simulink model "simu_21uec072"  (R2022b)
settings: Solver=VariableStepAuto  StartTime=0.0  StopTime=0  RelTol=1e-3
settings Model: Creator=DSP-35  LastModifiedBy=DSP-35

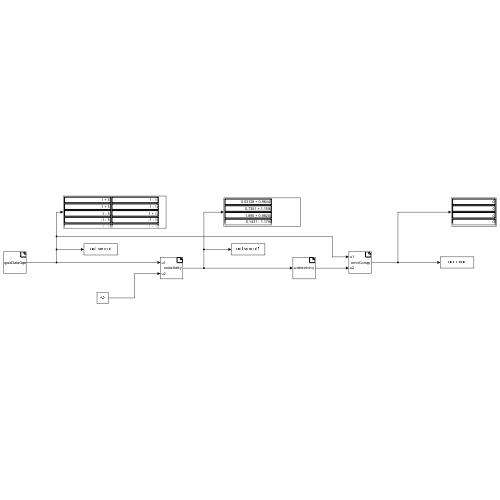
[thumbnail: Simulink's stored preview of the top-level diagram]
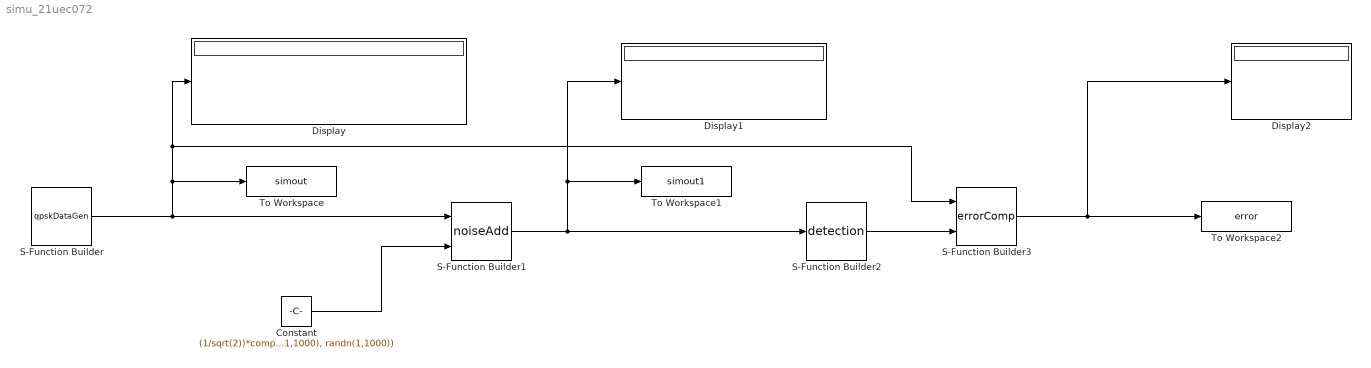
== system simu_21uec072 ==
  Constant : Constant  Value=(1/sqrt(2))*complex(randn(1,1000), randn(1,1000))
  Display : Display
  Display1 : Display
  Display2 : Display
  S-Function Builder : S-Function  FunctionName=qpskDataGen  SFunctionModules=qpskDataGen_wrapper.c  SFunctionDeploymentMode=off  EnableBusSupport=off  mask(S-Function Builder){}
      mask help: Simulink:masks:SFunctionBuilder_MD
      mask init:
      | val = [[.9  0.75 0.75 1 1 .9 .9 1]',[1 1 0.75 0.75 .9 .9 1 .9]'];try , sys = get_param(gcb,'SfunBuilderFcnName');if isempty(sys), sys = get_param(gcb,'FunctionName'); end,catch, sys = get_param(gcb,'FunctionName'); end
      settings: CopyFcn=set_param(gcbh,'LinkStatus','none')  OpenFcn=sfunctionwizard(gcbh)
      mask Display:
      | plot(val(:,1),val(:,2))
      | disp(sys)
      | port_label('output',1,'y')
  S-Function Builder1 : S-Function  FunctionName=noiseAdd  SFunctionModules=noiseAdd_wrapper.c  SFunctionDeploymentMode=off  EnableBusSupport=off  mask(S-Function Builder){}
      mask help: Simulink:masks:SFunctionBuilder_MD
      mask init: same as simu_21uec072/S-Function Builder
      settings: CopyFcn=set_param(gcbh,'LinkStatus','none')  OpenFcn=sfunctionwizard(gcbh)
      mask Display:
      | plot(val(:,1),val(:,2))
      | disp(sys)
      | port_label('input',1,'u1')
      | port_label('input',2,'u2')
      | port_label('output',1,'y')
  S-Function Builder2 : S-Function  FunctionName=detection  SFunctionModules=detection_wrapper.c  SFunctionDeploymentMode=off  EnableBusSupport=off  mask(S-Function Builder){}
      mask help: Simulink:masks:SFunctionBuilder_MD
      mask init: same as simu_21uec072/S-Function Builder
      settings: CopyFcn=set_param(gcbh,'LinkStatus','none')  OpenFcn=sfunctionwizard(gcbh)
      mask Display:
      | plot(val(:,1),val(:,2))
      | disp(sys)
      | port_label('input',1,'u')
      | port_label('output',1,'y')
  S-Function Builder3 : S-Function  FunctionName=errorComp  SFunctionModules=errorComp_wrapper.c  SFunctionDeploymentMode=off  EnableBusSupport=off  mask(S-Function Builder){}
      mask help: Simulink:masks:SFunctionBuilder_MD
      mask init: same as simu_21uec072/S-Function Builder
      settings: CopyFcn=set_param(gcbh,'LinkStatus','none')  OpenFcn=sfunctionwizard(gcbh)
      mask Display:
      | plot(val(:,1),val(:,2))
      | disp(sys)
      | port_label('input',1,'u1')
      | port_label('input',2,'u2')
      | port_label('output',1,'y')
  To Workspace : ToWorkspace  VariableName=simout  SampleTime=-1
      settings: Save2DSignal=2-D array (concatenate along first dimension)
  To Workspace1 : ToWorkspace  VariableName=simout1  SampleTime=-1
      settings: Save2DSignal=2-D array (concatenate along first dimension)
  To Workspace2 : ToWorkspace  VariableName=error  SampleTime=-1
      settings: Save2DSignal=2-D array (concatenate along first dimension)
  wires:
  S-Function Builder/1 -> Display/1, S-Function Builder3/1, To Workspace/1, S-Function Builder1/1
  Constant/1 -> S-Function Builder1/2
  S-Function Builder1/1 -> Display1/1, To Workspace1/1, S-Function Builder2/1
  S-Function Builder2/1 -> S-Function Builder3/2
  S-Function Builder3/1 -> Display2/1, To Workspace2/1
